simulink model "s_0303main"  (R2021a)
settings: Solver=FixedStepAuto  StartTime=0.0  StopTime=T_sim  FixedStep=dt  RelTol=1e-3
settings Model: Creator=paolo  LastModifiedBy=paolo

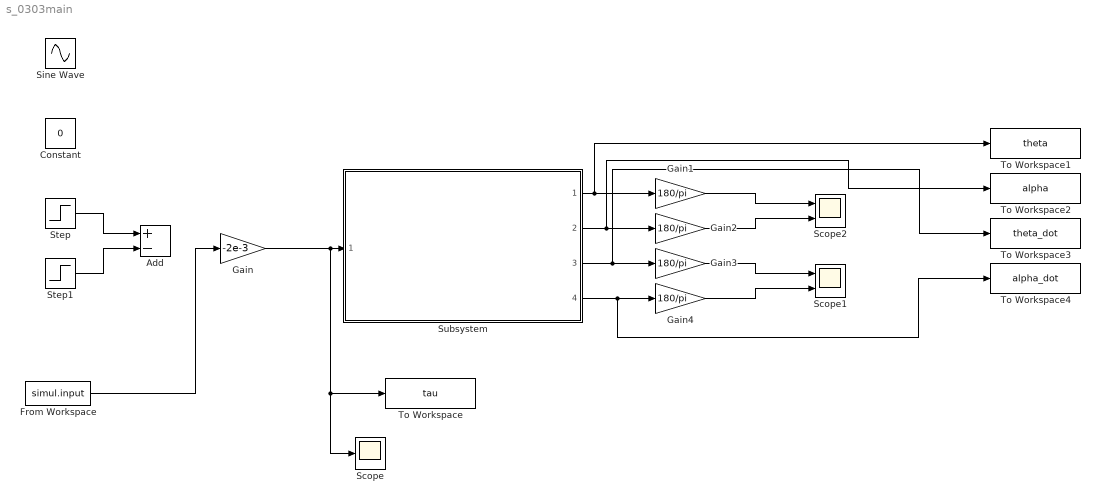
== system s_0303main ==
  Add : Sum  Inputs=+-
  Constant : Constant  Value=0
  From Workspace : FromWorkspace  VariableName=simul.input
  Gain : Gain  Gain=-2e-3
  Gain{1..4} (4 alike) : Gain  Gain=180/pi
  Scope : Scope
  Scope1 : Scope  NumInputPorts=2
  Scope2 : Scope  NumInputPorts=2
  Sine Wave : Sin  Frequency=2*2*pi  SampleTime=0
  Step : Step  SampleTime=0
  Step1 : Step  Time=2  SampleTime=0
  Subsystem : Subsystem  ReferencedSubsystem=s_0303simulator  th_0=0  al_0=0  th_dot_0=0  al_dot_0=0
  To Workspace : ToWorkspace  VariableName=tau  SampleTime=-1
  To Workspace1 : ToWorkspace  VariableName=theta  SampleTime=-1
  To Workspace2 : ToWorkspace  VariableName=alpha  SampleTime=-1
  To Workspace3 : ToWorkspace  VariableName=theta_dot  SampleTime=-1
  To Workspace4 : ToWorkspace  VariableName=alpha_dot  SampleTime=-1
  wires:
  Step/1 -> Add/1
  Step1/1 -> Add/2
  Subsystem/1 -> To Workspace1/1, Gain1/1
  Subsystem/2 -> To Workspace2/1, Gain2/1
  Gain1/1 -> Scope2/1
  Gain2/1 -> Scope2/2
  From Workspace/1 -> Gain/1
  Subsystem/4 -> To Workspace4/1, Gain4/1
  Gain4/1 -> Scope1/2
  Subsystem/3 -> To Workspace3/1, Gain3/1
  Gain3/1 -> Scope1/1
  Gain/1 -> Scope/1, To Workspace/1, Subsystem/1
